simulink library "util_mass_prop_lib"  (R2014b)
settings: Solver=ode45  StartTime=0.0  StopTime=10.0  RelTol=1e-3
libraries: util_mass_prop_lib x5, util_info_lib x4
settings Model: Creator=Mark Agbayani  LastModifiedBy=mstewart

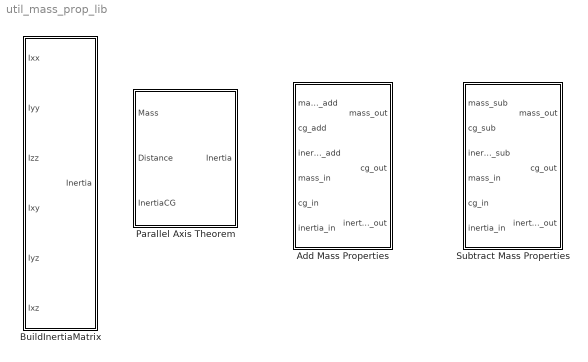
== system util_mass_prop_lib ==
  Add Mass Properties : Subsystem
      mask Display:
      | color('blue')
      | text(0.05,0.02,'MoonEx',...
      |  	'HorizontalAlignment','Left',...
      | 	'VerticalAlignment','bottom')
  BuildInertiaMatrix : Subsystem
      mask Display:
      | color('blue')
      | text(0.05,0.02,'MoonEx',...
      |  	'HorizontalAlignment','Left',...
      | 	'VerticalAlignment','bottom')
  Parallel Axis Theorem : Subsystem
      mask Display:
      | color('blue')
      | text(0.05,0.02,'MoonEx',...
      |  	'HorizontalAlignment','Left',...
      | 	'VerticalAlignment','bottom')
  Subtract Mass Properties : Subsystem
      mask Display:
      | color('blue')
      | text(0.05,0.02,'MoonEx',...
      |  	'HorizontalAlignment','Left',...
      | 	'VerticalAlignment','bottom')

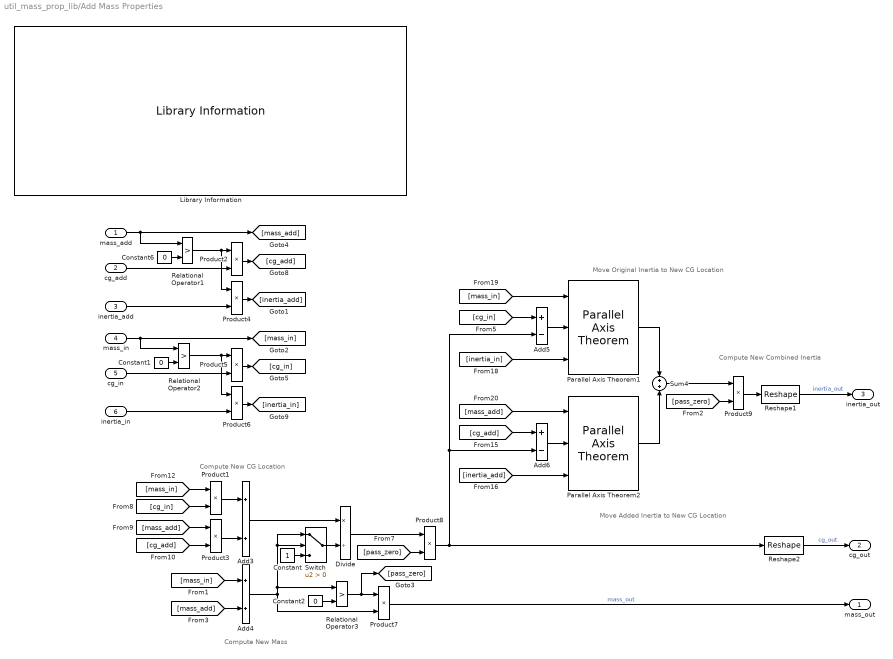
== system util_mass_prop_lib/Add Mass Properties ==
  note: Compute New CG Location
  note: Compute New Mass
  note: Move Original Inertia to New CG Location
  note: Move Added Inertia to New CG Location
  note: Compute New
      | Combined Inertia
  mass_add : Inport
  cg_add : Inport  Port=2
  inertia_add : Inport  Port=3
  mass_in : Inport  Port=4
  cg_in : Inport  Port=5
  inertia_in : Inport  Port=6
  Add3 : Sum
  Add4 : Sum
  Add5 : Sum  Inputs=+-
  Add6 : Sum  Inputs=+-
  Constant : Constant
  Constant1 : Constant  Value=0
  Constant2 : Constant  Value=0
  Constant6 : Constant  Value=0
  Divide : Product  Inputs=*/
  Library Information : util_info_lib/Library Information  owner='NONE'
  Parallel Axis Theorem1 : util_mass_prop_lib/Parallel Axis Theorem  SystemSampleTime=-1
  Parallel Axis Theorem2 : util_mass_prop_lib/Parallel Axis Theorem  SystemSampleTime=-1
  Product{1..9} (9 alike) : Product  RndMeth=Zero
  Relational Operator1 : RelationalOperator  Operator=>  OutDataTypeStr=float('double')
  Relational Operator2 : RelationalOperator  Operator=>  OutDataTypeStr=float('double')
  Relational Operator3 : RelationalOperator  Operator=>  OutDataTypeStr=float('double')
  Reshape1 : Reshape  OutputDimensionality=Customize  OutputDimensions=[3,3]
  Reshape2 : Reshape  OutputDimensions=[3,3]
  Sum4 : Sum  Inputs=+|+
  Switch : Switch  Criteria=u2 > Threshold
  mass_out : Outport
  cg_out : Outport  Port=2
  inertia_out : Outport  Port=3
  wires:
  mass_add/1 -> [mass_add], Relational Operator1/1
  [mass_add] -> Add4/2
  [mass_in] -> Add4/1
  [mass_in] -> Product1/1
  [cg_in] -> Product1/2
  Product1/1 -> Add3/1
  Product3/1 -> Add3/2
  [mass_add] -> Product3/1
  [cg_add] -> Product3/2
  Add3/1 -> Divide/1
  [cg_in] -> Add5/1
  [mass_in] -> Parallel Axis Theorem1/1
  Add5/1 -> Parallel Axis Theorem1/2
  [inertia_in] -> Parallel Axis Theorem1/3
  [mass_add] -> Parallel Axis Theorem2/1
  Add6/1 -> Parallel Axis Theorem2/2
  [cg_add] -> Add6/1
  Parallel Axis Theorem1/1 -> Sum4/1
  Parallel Axis Theorem2/1 -> Sum4/2
  [inertia_add] -> Parallel Axis Theorem2/3
  Relational Operator1/1 -> Product2/1, Product4/1
  Product2/1 -> [cg_add]
  cg_add/1 -> Product2/2
  Product4/1 -> [inertia_add]
  inertia_add/1 -> Product4/2
  Relational Operator2/1 -> Product6/1, Product5/1
  cg_in/1 -> Product5/2
  inertia_in/1 -> Product6/2
  mass_in/1 -> [mass_in], Relational Operator2/1
  Product5/1 -> [cg_in]
  Product6/1 -> [inertia_in]
  Relational Operator3/1 -> [pass_zero], Product7/1
  [pass_zero] -> Product8/2
  Divide/1 -> Product8/1
  Add4/1 -> Product7/2, Switch/2, Switch/1, Relational Operator3/1
  Product7/1 -> mass_out/1  "mass_out"
  Switch/1 -> Divide/2
  Constant/1 -> Switch/3
  Product8/1 -> Add6/2, Add5/2, Reshape2/1
  [pass_zero] -> Product9/2
  Sum4/1 -> Product9/1
  Product9/1 -> Reshape1/1
  Reshape1/1 -> inertia_out/1  "inertia_out"
  Reshape2/1 -> cg_out/1  "cg_out"
  Constant6/1 -> Relational Operator1/2
  Constant1/1 -> Relational Operator2/2
  Constant2/1 -> Relational Operator3/2

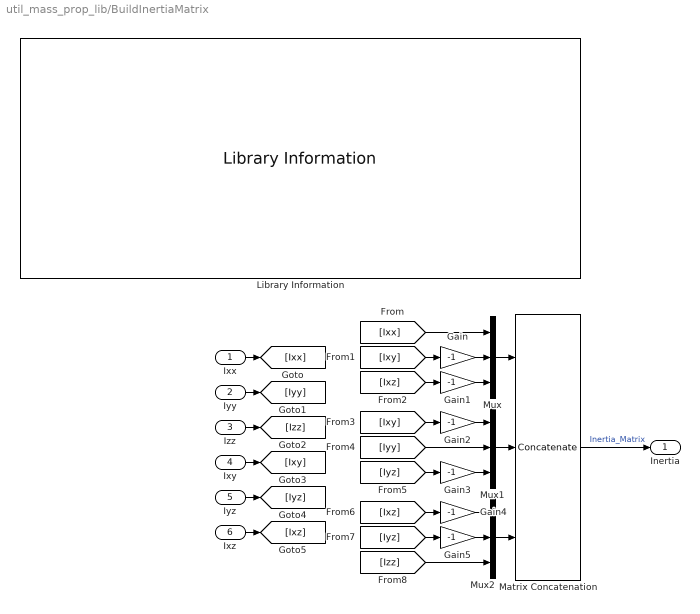
== system util_mass_prop_lib/BuildInertiaMatrix ==
  Ixx : Inport
  Iyy : Inport  Port=2
  Izz : Inport  Port=3
  Ixy : Inport  Port=4
  Iyz : Inport  Port=5
  Ixz : Inport  Port=6
  Gain{,1..5} (6 alike) : Gain  Gain=-1  SaturateOnIntegerOverflow=on  OutDataTypeStr=Inherit: Same as input  ParamDataTypeStr=Inherit: Same as input
  Library Information : util_info_lib/Library Information  owner='NONE'
  Matrix Concatenation : Concatenate  NumInputs=3  Mode=Multidimensional array  ConcatenateDimension=2
  Mux : Mux  Inputs=3
  Mux1 : Mux  Inputs=3
  Mux2 : Mux  Inputs=3
  Inertia : Outport
  wires:
  Ixx/1 -> [Ixx]
  Iyy/1 -> [Iyy]
  Izz/1 -> [Izz]
  [Ixx] -> Mux/1
  [Ixy] -> Gain/1
  [Ixz] -> Gain1/1
  Mux/1 -> Matrix Concatenation/1
  Matrix Concatenation/1 -> Inertia/1  "Inertia_Matrix"
  Ixy/1 -> [Ixy]
  Iyz/1 -> [Iyz]
  Ixz/1 -> [Ixz]
  Gain/1 -> Mux/2
  Gain1/1 -> Mux/3
  [Iyy] -> Mux1/2
  [Iyz] -> Gain3/1
  Gain3/1 -> Mux1/3
  [Ixy] -> Gain2/1
  Gain2/1 -> Mux1/1
  Mux1/1 -> Matrix Concatenation/2
  [Izz] -> Mux2/3
  [Ixz] -> Gain4/1
  Gain4/1 -> Mux2/1
  Mux2/1 -> Matrix Concatenation/3
  [Iyz] -> Gain5/1
  Gain5/1 -> Mux2/2

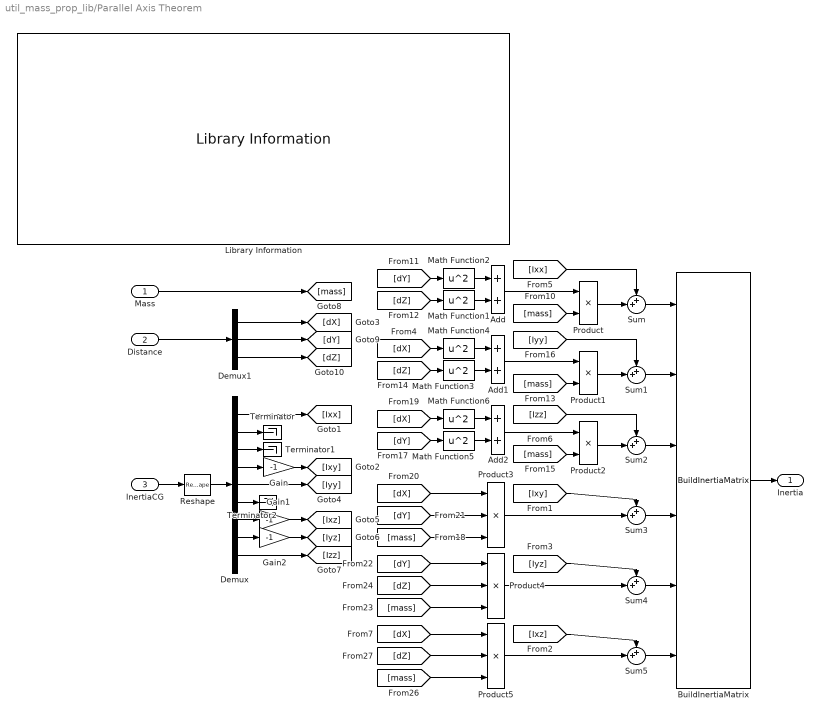
== system util_mass_prop_lib/Parallel Axis Theorem ==
  Mass : Inport
  Distance : Inport  Port=2
  InertiaCG : Inport  Port=3
  Add : Sum
  Add1 : Sum
  Add2 : Sum
  BuildInertiaMatrix : util_mass_prop_lib/BuildInertiaMatrix  SystemSampleTime=-1
  Demux : Demux  Outputs=9
  Demux1 : Demux  Outputs=3
  Gain : Gain  Gain=-1  SaturateOnIntegerOverflow=on  OutDataTypeStr=Inherit: Same as input  ParamDataTypeStr=Inherit: Same as input
  Gain1 : Gain  Gain=-1  SaturateOnIntegerOverflow=on  OutDataTypeStr=Inherit: Same as input  ParamDataTypeStr=Inherit: Same as input
  Gain2 : Gain  Gain=-1  SaturateOnIntegerOverflow=on  OutDataTypeStr=Inherit: Same as input  ParamDataTypeStr=Inherit: Same as input
  Library Information : util_info_lib/Library Information  owner='NONE'
  Math Function{1..6} (6 alike) : Math  Operator=square  SaturateOnIntegerOverflow=on
  Product : Product  RndMeth=Zero
  Product1 : Product  RndMeth=Zero
  Product2 : Product  RndMeth=Zero
  Product3 : Product  Inputs=3  RndMeth=Zero
  Product4 : Product  Inputs=3  RndMeth=Zero
  Product5 : Product  Inputs=3  RndMeth=Zero
  Reshape : Reshape
  Sum{,1..5} (6 alike) : Sum  Inputs=++|
  Terminator : Terminator
  Terminator1 : Terminator
  Terminator2 : Terminator
  Inertia : Outport
  wires:
  BuildInertiaMatrix/1 -> Inertia/1
  InertiaCG/1 -> Reshape/1
  Reshape/1 -> Demux/1
  Demux/1 -> [Ixx]
  Demux/2 -> Terminator/1
  Demux/3 -> Terminator1/1
  Demux/4 -> Gain/1
  Demux/5 -> [Iyy]
  Demux/6 -> Terminator2/1
  Demux/7 -> Gain1/1
  Demux/8 -> Gain2/1
  Demux/9 -> [Izz]
  Mass/1 -> [mass]
  Distance/1 -> Demux1/1
  Demux1/1 -> [dX]
  Demux1/2 -> [dY]
  Demux1/3 -> [dZ]
  Math Function2/1 -> Add/1
  Math Function1/1 -> Add/2
  [dY] -> Math Function2/1
  [dZ] -> Math Function1/1
  Add/1 -> Product/1
  [mass] -> Product/2
  Product/1 -> Sum/2
  Sum/1 -> BuildInertiaMatrix/1
  [Ixx] -> Sum/1
  Gain/1 -> [Ixy]
  Gain1/1 -> [Ixz]
  Gain2/1 -> [Iyz]
  Math Function4/1 -> Add1/1
  Math Function3/1 -> Add1/2
  [dX] -> Math Function4/1
  [dZ] -> Math Function3/1
  Add1/1 -> Product1/1
  [mass] -> Product1/2
  Product1/1 -> Sum1/2
  [Iyy] -> Sum1/1
  Sum1/1 -> BuildInertiaMatrix/2
  Math Function6/1 -> Add2/1
  Math Function5/1 -> Add2/2
  [dX] -> Math Function6/1
  [dY] -> Math Function5/1
  Add2/1 -> Product2/1
  [mass] -> Product2/2
  Product2/1 -> Sum2/2
  [Izz] -> Sum2/1
  Sum2/1 -> BuildInertiaMatrix/3
  [Ixy] -> Sum3/1
  Product3/1 -> Sum3/2
  [dX] -> Product3/1
  [dY] -> Product3/2
  [mass] -> Product3/3
  Sum3/1 -> BuildInertiaMatrix/4
  [Iyz] -> Sum4/1
  Product4/1 -> Sum4/2
  [dY] -> Product4/1
  [dZ] -> Product4/2
  [mass] -> Product4/3
  Sum4/1 -> BuildInertiaMatrix/5
  [Ixz] -> Sum5/1
  Product5/1 -> Sum5/2
  [dX] -> Product5/1
  [dZ] -> Product5/2
  [mass] -> Product5/3
  Sum5/1 -> BuildInertiaMatrix/6

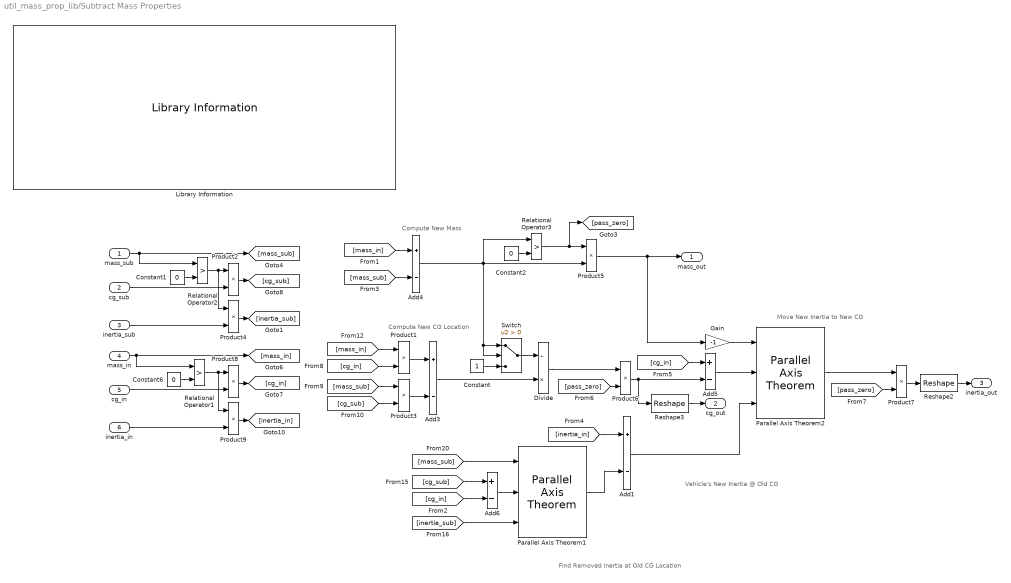
== system util_mass_prop_lib/Subtract Mass Properties ==
  note: Find Removed Inertia at Old CG Location
  note: Move New Inertia to New CG
  note: Compute New Mass
  note: Compute New CG Location
  note: Vehicle's New
      | Inertia @ Old CG
  mass_sub : Inport
  cg_sub : Inport  Port=2
  inertia_sub : Inport  Port=3
  mass_in : Inport  Port=4
  cg_in : Inport  Port=5
  inertia_in : Inport  Port=6
  Add{1,3..6} (5 alike) : Sum  Inputs=+-
  Constant : Constant
  Constant1 : Constant  Value=0
  Constant2 : Constant  Value=0
  Constant6 : Constant  Value=0
  Divide : Product  Inputs=/*
  Gain : Gain  Gain=-1  SaturateOnIntegerOverflow=on  OutDataTypeStr=Inherit: Same as input  ParamDataTypeStr=Inherit: Same as input
  Library Information : util_info_lib/Library Information  owner='NONE'
  Parallel Axis Theorem1 : util_mass_prop_lib/Parallel Axis Theorem  SystemSampleTime=-1
  Parallel Axis Theorem2 : util_mass_prop_lib/Parallel Axis Theorem  SystemSampleTime=-1
  Product{1..9} (9 alike) : Product  RndMeth=Zero
  Relational Operator1 : RelationalOperator  Operator=>  OutDataTypeStr=float('double')
  Relational Operator2 : RelationalOperator  Operator=>  OutDataTypeStr=float('double')
  Relational Operator3 : RelationalOperator  Operator=>  OutDataTypeStr=float('double')
  Reshape2 : Reshape  OutputDimensionality=Customize  OutputDimensions=[3,3]
  Reshape3 : Reshape  OutputDimensions=[3,3]
  Switch : Switch  Criteria=u2 > Threshold
  mass_out : Outport
  cg_out : Outport  Port=2
  inertia_out : Outport  Port=3
  wires:
  [cg_sub] -> Add6/1
  [inertia_sub] -> Parallel Axis Theorem1/3
  Add6/1 -> Parallel Axis Theorem1/2
  [mass_sub] -> Parallel Axis Theorem1/1
  Add1/1 -> Parallel Axis Theorem2/3
  Add5/1 -> Parallel Axis Theorem2/2
  Gain/1 -> Parallel Axis Theorem2/1
  [cg_in] -> Add5/1
  Add3/1 -> Divide/2
  [cg_sub] -> Product3/2
  [mass_sub] -> Product3/1
  Product3/1 -> Add3/2
  Product1/1 -> Add3/1
  [cg_in] -> Product1/2
  [mass_in] -> Product1/1
  [mass_in] -> Add4/1
  [mass_sub] -> Add4/2
  Add4/1 -> Product5/2, Switch/1, Switch/2, Relational Operator3/1
  mass_sub/1 -> [mass_sub], Relational Operator2/1
  [cg_in] -> Add6/2
  [inertia_in] -> Add1/1
  Divide/1 -> Product6/1
  Parallel Axis Theorem1/1 -> Add1/2
  Relational Operator2/1 -> Product4/1, Product2/1
  Product2/1 -> [cg_sub]
  Product4/1 -> [inertia_sub]
  inertia_sub/1 -> Product4/2
  cg_sub/1 -> Product2/2
  Relational Operator3/1 -> Product5/1, [pass_zero]
  Product5/1 -> mass_out/1, Gain/1
  Switch/1 -> Divide/1
  Constant/1 -> Switch/3
  [pass_zero] -> Product6/2
  [pass_zero] -> Product7/2
  Parallel Axis Theorem2/1 -> Product7/1
  Product7/1 -> Reshape2/1
  Relational Operator1/1 -> Product8/1, Product9/1
  cg_in/1 -> Product8/2
  inertia_in/1 -> Product9/2
  mass_in/1 -> [mass_in], Relational Operator1/1
  Product8/1 -> [cg_in]
  Product9/1 -> [inertia_in]
  Product6/1 -> Reshape3/1, Add5/2
  Reshape3/1 -> cg_out/1
  Reshape2/1 -> inertia_out/1
  Constant6/1 -> Relational Operator1/2
  Constant1/1 -> Relational Operator2/2
  Constant2/1 -> Relational Operator3/2
